simulink model "modelsimulator"  (R2023b)
settings: Solver=VariableStepAuto  StartTime=0.0  StopTime=185  FixedStep=0.0002  RelTol=1e-3
values from neighbouring files (symbols this model uses):
  eta_init = [0 0 0 0 0 0]    [Linearization_validation.m]    (also in ROV_simulation_init.m = [radius 0 0 0 0 -pi/2])
  K_full = lqr(linsysROV_lqr,Q,R)    [ROV_simulation_init.m]
  K_reduced = lqr(linsysROV_lqr_reduced_disc,Q,R)    [ROV_simulation_init.m]
  omega = 0.0174532925*5    (= 0.0872664625)    [ROV_simulation_init.m]
  p = [-125.691529893755	-8.50647884753240	275.922008410927	13.4112646958028	-226.567986780204	-3.28875901062827	118.657519470084	6.62648580653865	14.9826070833980	0.00]    [ROV_simulation_init.m]
  PID_phi = [11.6676, 5.8503, -12.3688, 0.025226,34]    [ROV_simulation_init.m]
  PID_psi = [11.3054, 1.000, -3.8005, 0.087502,30]    [ROV_simulation_init.m]
  PID_theta = [10.2974, 5.9702, -15.653, 0.016423,19]    [ROV_simulation_init.m]
  PID_x = [500.411, 30.5093, -500.8638, 0.032394,110]    [ROV_simulation_init.m]
  PID_y = [500.7275, 20.1075, -500.8002, 0.019369,110]    [ROV_simulation_init.m]
  PID_z = [500.7655, 25.0859, -500.5557, 0.026709,158]    [ROV_simulation_init.m]
  radius = 5    [ROV_simulation_init.m]
  ROV = initializeModelMatrices(m,I,COG,l,w,h,Thrusters)    [CreateGramianROV.m]    (also in CreateROVLin.m = initializeModelMatrices(m, I, COB, dim, BlueROVHeavy); Eigenvalue_tracking.m = initializeModelMatrices(m, I, COB,dim,0); Linearization_validation.m = initializeModelMatrices(m, I, COB,dim,0); ROV_simulation_init.m = initializeModelMatrices(m, Inertia, COB, dim, BlueROVHeavy))
  T_inv = ROV.T'/(ROV.T*ROV.T')    [ROV_simulation_init.m]
  ThrusterVoltage = 14    [ROV_simulation_init.m]
  v_init = [3 0 0 0 0 0]    [Linearization_validation.m]    (also in ROV_simulation_init.m = [omega omega z_rate 0 0 omega])
  z_rate = 0.1    [ROV_simulation_init.m]
libraries: simulink x60
(part 2 of 3)

== system modelsimulator/LQR_full/Subsystem ==
  eta_ref : Inport
  Cos : Trigonometry  Operator=cos
  Demux : Demux  Outputs=6
  Gain : Gain  Gain=1.32
  Gain1 : Gain  Gain=1.32
  Mux : Mux  Inputs=6
  Product : Product
  Sin : Trigonometry
  Sin1 : Trigonometry
  Out1 : Outport
  wires:
  Demux/4 -> Sin/1
  Mux/1 -> Out1/1
  Demux/5 -> Sin1/1, Cos/1
  Gain/1 -> Mux/4
  Product/1 -> Gain/1
  Sin/1 -> Product/1
  Cos/1 -> Product/2
  Gain1/1 -> Mux/5
  Sin1/1 -> Gain1/1
  eta_ref/1 -> Demux/1

== system modelsimulator/LQR_full/Tau_body ==
  Tau : Inport
  Pos : Inport  Port=2
  Demux : Demux  Outputs=6
  Demux1 : Demux  Outputs=6
  InvNED : MATLAB Function  TreatAsAtomicUnit=on
  Mux : Mux  Inputs=6
  Tau_b : Outport
  wires:
  Demux/6 -> InvNED/6(Tau6)
  Demux/5 -> InvNED/5(Tau5)
  Demux/3 -> InvNED/3(Tau3)
  Demux/4 -> InvNED/4(Tau4)
  Demux/2 -> InvNED/2(Tau2)
  Demux/1 -> InvNED/1(Tau1)
  Tau/1 -> Demux/1
  Demux1/1 -> InvNED/7(x)
  Demux1/2 -> InvNED/8(y)
  Demux1/3 -> InvNED/9(z)
  Demux1/4 -> InvNED/10(phi)
  Demux1/5 -> InvNED/11(theta)
  Demux1/6 -> InvNED/12(pzi)
  InvNED/1(x_dot) -> Mux/1
  InvNED/2(y_dot) -> Mux/2
  InvNED/3(z_dot) -> Mux/3
  InvNED/4(phi_dot) -> Mux/4
  InvNED/5(theta_dot) -> Mux/5
  InvNED/6(pzi_dot) -> Mux/6
  Mux/1 -> Tau_b/1
  Pos/1 -> Demux1/1

== system modelsimulator/LQR_reduced/Force allocation ==
  Tau : Inport
  1-D Lookup Table : Lookup_n-D  NumberOfTableDimensions=1  BreakpointsForDimension1=polyval(p,[-1:0.1:1])  Table=[-1:0.1:1]  InternalRulePriority=Speed  RndMeth=Simplest
  Constant7 : Constant  Value=T_inv
  Matrix Multiply : Product  Multiplication=Matrix(*)
  u : Outport
  wires:
  Constant7/1 -> Matrix Multiply/1
  Tau/1 -> Matrix Multiply/2
  Matrix Multiply/1 -> 1-D Lookup Table/1
  1-D Lookup Table/1 -> u/1

== system modelsimulator/LQR_reduced/Subsystem ==
  eta_ref : Inport
  Cos : Trigonometry  Operator=cos
  Demux : Demux  Outputs=6
  Gain : Gain  Gain=1.32
  Gain1 : Gain  Gain=1.32
  Mux : Mux  Inputs=6
  Product : Product
  Sin : Trigonometry
  Sin1 : Trigonometry
  Out1 : Outport
  wires:
  Demux/4 -> Sin/1
  Mux/1 -> Out1/1
  Demux/5 -> Sin1/1, Cos/1
  Gain/1 -> Mux/4
  Product/1 -> Gain/1
  Sin/1 -> Product/1
  Cos/1 -> Product/2
  Gain1/1 -> Mux/5
  Sin1/1 -> Gain1/1
  eta_ref/1 -> Demux/1

== system modelsimulator/PID/Force allocation ==
  Tau : Inport
  1-D Lookup Table : Lookup_n-D  NumberOfTableDimensions=1  BreakpointsForDimension1=polyval(p,[-1:0.1:1])  Table=[-1:0.1:1]  InternalRulePriority=Speed  RndMeth=Simplest
  Constant7 : Constant  Value=T_inv
  Matrix Multiply : Product  Multiplication=Matrix(*)
  u : Outport
  wires:
  Constant7/1 -> Matrix Multiply/1
  Tau/1 -> Matrix Multiply/2
  Matrix Multiply/1 -> 1-D Lookup Table/1
  1-D Lookup Table/1 -> u/1

== system modelsimulator/PID/G1 ==
  ref : Inport
  position : Inport  Port=2
  Derivative : Derivative
  Filter : TransferFcn  Denominator=[Tf 1]
  Gain : Gain  Gain=Kc
  Gain1 : Gain  Gain=Ki
  Gain2 : Gain  Gain=Kd
  Integrator : Integrator  InitialCondition=Arb_pnk  LimitOutput=on  UpperSaturationLimit=umax  LowerSaturationLimit=-umax
  Sum : Sum  Inputs=||+++
  Sum1 : Sum  Inputs=|+-
  u : Outport
  wires:
  Gain2/1 -> Derivative/1
  Gain/1 -> Sum/1
  Derivative/1 -> Sum/3
  Integrator/1 -> Sum/2
  Gain1/1 -> Integrator/1
  Filter/1 -> Gain2/1
  Sum/1 -> u/1
  Sum1/1 -> Gain1/1, Gain/1
  ref/1 -> Sum1/1
  position/1 -> Filter/1, Sum1/2

== system modelsimulator/PID/G2 ==
  ref : Inport
  position : Inport  Port=2
  Derivative : Derivative
  Filter : TransferFcn  Denominator=[Tf 1]
  Gain : Gain  Gain=Kc
  Gain1 : Gain  Gain=Ki
  Gain2 : Gain  Gain=Kd
  Integrator : Integrator  InitialCondition=Arb_pnk  LimitOutput=on  UpperSaturationLimit=umax  LowerSaturationLimit=-umax
  Sum : Sum  Inputs=||+++
  Sum1 : Sum  Inputs=|+-
  u : Outport
  wires:
  position/1 -> Sum1/2, Filter/1
  ref/1 -> Sum1/1
  Sum1/1 -> Gain/1, Gain1/1
  Sum/1 -> u/1
  Filter/1 -> Gain2/1
  Gain1/1 -> Integrator/1
  Integrator/1 -> Sum/2
  Derivative/1 -> Sum/3
  Gain/1 -> Sum/1
  Gain2/1 -> Derivative/1

== system modelsimulator/PID/G3 ==
  ref : Inport
  position : Inport  Port=2
  Derivative : Derivative
  Filter : TransferFcn  Denominator=[Tf 1]
  Gain : Gain  Gain=Kc
  Gain1 : Gain  Gain=Ki
  Gain2 : Gain  Gain=Kd
  Integrator : Integrator  InitialCondition=Arb_pnk  LimitOutput=on  UpperSaturationLimit=umax  LowerSaturationLimit=-umax
  Sum : Sum  Inputs=||+++
  Sum1 : Sum  Inputs=|+-
  u : Outport
  wires:
  Gain2/1 -> Derivative/1
  Gain/1 -> Sum/1
  Derivative/1 -> Sum/3
  Integrator/1 -> Sum/2
  Gain1/1 -> Integrator/1
  Filter/1 -> Gain2/1
  Sum/1 -> u/1
  Sum1/1 -> Gain1/1, Gain/1
  ref/1 -> Sum1/1
  position/1 -> Filter/1, Sum1/2

== system modelsimulator/PID/G4 ==
  ref : Inport
  position : Inport  Port=2
  Derivative : Derivative
  Filter : TransferFcn  Denominator=[Tf 1]
  Gain : Gain  Gain=Kc
  Gain1 : Gain  Gain=Ki
  Gain2 : Gain  Gain=Kd
  Integrator : Integrator  InitialCondition=Arb_pnk  LimitOutput=on  UpperSaturationLimit=umax  LowerSaturationLimit=-umax
  Sum : Sum  Inputs=||+++
  Sum1 : Sum  Inputs=|+-
  u : Outport
  wires:
  position/1 -> Sum1/2, Filter/1
  ref/1 -> Sum1/1
  Sum1/1 -> Gain/1, Gain1/1
  Sum/1 -> u/1
  Filter/1 -> Gain2/1
  Gain1/1 -> Integrator/1
  Integrator/1 -> Sum/2
  Derivative/1 -> Sum/3
  Gain/1 -> Sum/1
  Gain2/1 -> Derivative/1

== system modelsimulator/PID/G5 ==
  ref : Inport
  position : Inport  Port=2
  Derivative : Derivative
  Filter : TransferFcn  Denominator=[Tf 1]
  Gain : Gain  Gain=Kc
  Gain1 : Gain  Gain=Ki
  Gain2 : Gain  Gain=Kd
  Integrator : Integrator  InitialCondition=Arb_pnk  LimitOutput=on  UpperSaturationLimit=umax  LowerSaturationLimit=-umax
  Sum : Sum  Inputs=||+++
  Sum1 : Sum  Inputs=|+-
  u : Outport
  wires:
  Gain2/1 -> Derivative/1
  Gain/1 -> Sum/1
  Derivative/1 -> Sum/3
  Integrator/1 -> Sum/2
  Gain1/1 -> Integrator/1
  Filter/1 -> Gain2/1
  Sum/1 -> u/1
  Sum1/1 -> Gain1/1, Gain/1
  ref/1 -> Sum1/1
  position/1 -> Filter/1, Sum1/2

== system modelsimulator/PID/G6 ==
  ref : Inport
  position : Inport  Port=2
  Derivative : Derivative
  Filter : TransferFcn  Denominator=[Tf 1]
  Gain : Gain  Gain=Kc
  Gain1 : Gain  Gain=Ki
  Gain2 : Gain  Gain=Kd
  Integrator : Integrator  InitialCondition=Arb_pnk  LimitOutput=on  UpperSaturationLimit=umax  LowerSaturationLimit=-umax
  Sum : Sum  Inputs=||+++
  Sum1 : Sum  Inputs=|+-
  u : Outport
  wires:
  position/1 -> Sum1/2, Filter/1
  ref/1 -> Sum1/1
  Sum1/1 -> Gain/1, Gain1/1
  Sum/1 -> u/1
  Filter/1 -> Gain2/1
  Gain1/1 -> Integrator/1
  Integrator/1 -> Sum/2
  Derivative/1 -> Sum/3
  Gain/1 -> Sum/1
  Gain2/1 -> Derivative/1

== system modelsimulator/PID/Tau_body ==
  Tau : Inport
  Pos : Inport  Port=2
  Demux : Demux  Outputs=6
  Demux1 : Demux  Outputs=6
  InvNED : MATLAB Function  TreatAsAtomicUnit=on
  Mux : Mux  Inputs=6
  Tau_b : Outport
  wires:
  Demux/6 -> InvNED/6(Tau6)
  Demux/5 -> InvNED/5(Tau5)
  Demux/3 -> InvNED/3(Tau3)
  Demux/4 -> InvNED/4(Tau4)
  Demux/2 -> InvNED/2(Tau2)
  Demux/1 -> InvNED/1(Tau1)
  Tau/1 -> Demux/1
  Demux1/1 -> InvNED/7(x)
  Demux1/2 -> InvNED/8(y)
  Demux1/3 -> InvNED/9(z)
  Demux1/4 -> InvNED/10(phi)
  Demux1/5 -> InvNED/11(theta)
  Demux1/6 -> InvNED/12(pzi)
  InvNED/1(x_dot) -> Mux/1
  InvNED/2(y_dot) -> Mux/2
  InvNED/3(z_dot) -> Mux/3
  InvNED/4(phi_dot) -> Mux/4
  InvNED/5(theta_dot) -> Mux/5
  InvNED/6(pzi_dot) -> Mux/6
  Mux/1 -> Tau_b/1
  Pos/1 -> Demux1/1

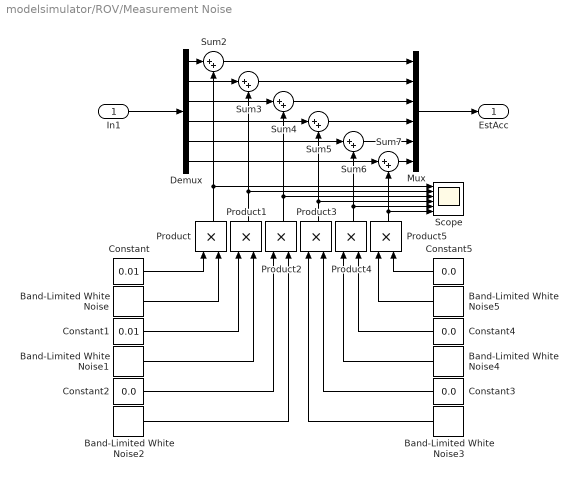
== system modelsimulator/ROV/Measurement Noise ==
  In1 : Inport
  Band-Limited White Noise : simulink/Sources/Band-Limited White Noise  Cov=0.00001  Ts=0.01  seed=[23341]  VectorParams1D=off
  Band-Limited White Noise1 : simulink/Sources/Band-Limited White Noise  Cov=0.00001  Ts=0.01  seed=[23342]  VectorParams1D=off
  Band-Limited White Noise2 : simulink/Sources/Band-Limited White Noise  Cov=0.00001  Ts=0.01  seed=[23343]  VectorParams1D=off
  Band-Limited White Noise3 : simulink/Sources/Band-Limited White Noise  Cov=0.00001  Ts=0.01  seed=[23344]  VectorParams1D=off
  Band-Limited White Noise4 : simulink/Sources/Band-Limited White Noise  Cov=0.00001  Ts=0.01  seed=[23345]  VectorParams1D=off
  Band-Limited White Noise5 : simulink/Sources/Band-Limited White Noise  Cov=0.00001  Ts=0.01  seed=[23346]  VectorParams1D=off
  Constant : Constant  Value=0.01
  Constant1 : Constant  Value=0.01
  Constant{2..5} (4 alike) : Constant  Value=0.0
  Demux : Demux  Outputs=6
  Mux : Mux  Inputs=6
  Product{,1..5} (6 alike) : Product
  Scope : Scope  NumInputPorts=6
  Sum{2..7} (6 alike) : Sum  Inputs=|++
  EstAcc : Outport
  wires:
  Product1/1 -> Scope/2, Sum3/2
  Sum3/1 -> Mux/2
  Demux/2 -> Sum3/1
  Product2/1 -> Scope/3, Sum4/2
  Product4/1 -> Scope/5, Sum6/2
  Band-Limited White Noise5/1 -> Product5/1
  Product5/1 -> Scope/6, Sum7/2
  Constant/1 -> Product/1
  Demux/5 -> Sum6/1
  Band-Limited White Noise1/1 -> Product1/2
  Sum7/1 -> Mux/6
  Product3/1 -> Scope/4, Sum5/2
  Product/1 -> Sum2/2, Scope/1
  Band-Limited White Noise/1 -> Product/2
  Demux/1 -> Sum2/1
  Sum5/1 -> Mux/4
  Sum2/1 -> Mux/1
  Sum4/1 -> Mux/3
  Demux/3 -> Sum4/1
  Band-Limited White Noise3/1 -> Product3/1
  Band-Limited White Noise2/1 -> Product2/2
  Demux/4 -> Sum5/1
  Sum6/1 -> Mux/5
  Mux/1 -> EstAcc/1
  Demux/6 -> Sum7/1
  Band-Limited White Noise4/1 -> Product4/1
  In1/1 -> Demux/1
  Constant1/1 -> Product1/1
  Constant2/1 -> Product2/1
  Constant3/1 -> Product3/2
  Constant4/1 -> Product4/2
  Constant5/1 -> Product5/2

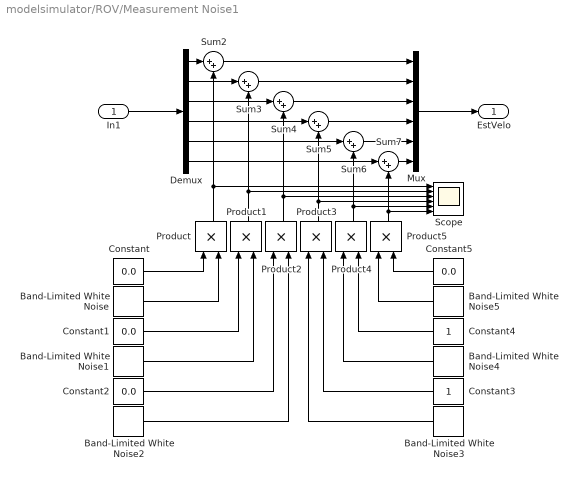
== system modelsimulator/ROV/Measurement Noise1 ==
  In1 : Inport
  Band-Limited White Noise : simulink/Sources/Band-Limited White Noise  Cov=0.00001  Ts=0.01  seed=[23341]  VectorParams1D=off
  Band-Limited White Noise1 : simulink/Sources/Band-Limited White Noise  Cov=0.00001  Ts=0.01  seed=[23342]  VectorParams1D=off
  Band-Limited White Noise2 : simulink/Sources/Band-Limited White Noise  Cov=0.00001  Ts=0.01  seed=[23343]  VectorParams1D=off
  Band-Limited White Noise3 : simulink/Sources/Band-Limited White Noise  Cov=0.00001  Ts=0.01  seed=[23344]  VectorParams1D=off
  Band-Limited White Noise4 : simulink/Sources/Band-Limited White Noise  Cov=0.00001  Ts=0.01  seed=[23345]  VectorParams1D=off
  Band-Limited White Noise5 : simulink/Sources/Band-Limited White Noise  Cov=0.00001  Ts=0.01  seed=[23346]  VectorParams1D=off
  Constant{,1..2,5} (4 alike) : Constant  Value=0.0
  Constant3 : Constant
  Constant4 : Constant
  Demux : Demux  Outputs=6
  Mux : Mux  Inputs=6
  Product{,1..5} (6 alike) : Product
  Scope : Scope  NumInputPorts=6
  Sum{2..7} (6 alike) : Sum  Inputs=|++
  EstVelo : Outport
  wires:
  Constant5/1 -> Product5/2
  Constant4/1 -> Product4/2
  Constant3/1 -> Product3/2
  Constant2/1 -> Product2/1
  Constant1/1 -> Product1/1
  In1/1 -> Demux/1
  Band-Limited White Noise4/1 -> Product4/1
  Demux/6 -> Sum7/1
  Mux/1 -> EstVelo/1
  Sum6/1 -> Mux/5
  Demux/4 -> Sum5/1
  Band-Limited White Noise2/1 -> Product2/2
  Band-Limited White Noise3/1 -> Product3/1
  Demux/3 -> Sum4/1
  Sum4/1 -> Mux/3
  Sum2/1 -> Mux/1
  Sum5/1 -> Mux/4
  Demux/1 -> Sum2/1
  Band-Limited White Noise/1 -> Product/2
  Product/1 -> Scope/1, Sum2/2
  Product3/1 -> Sum5/2, Scope/4
  Sum7/1 -> Mux/6
  Band-Limited White Noise1/1 -> Product1/2
  Demux/5 -> Sum6/1
  Constant/1 -> Product/1
  Product5/1 -> Sum7/2, Scope/6
  Band-Limited White Noise5/1 -> Product5/1
  Product4/1 -> Sum6/2, Scope/5
  Product2/1 -> Sum4/2, Scope/3
  Demux/2 -> Sum3/1
  Sum3/1 -> Mux/2
  Product1/1 -> Sum3/2, Scope/2

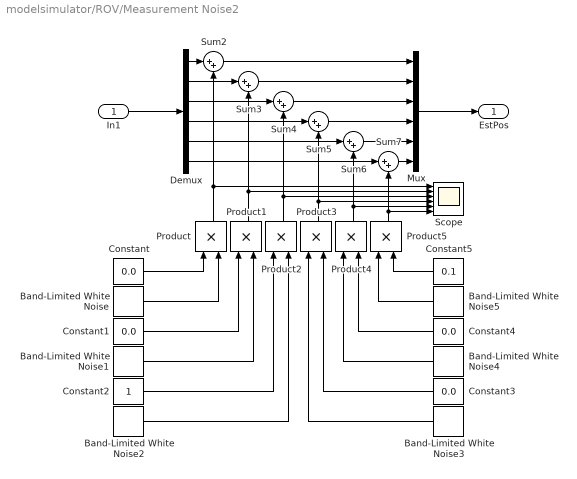
== system modelsimulator/ROV/Measurement Noise2 ==
  In1 : Inport
  Band-Limited White Noise : simulink/Sources/Band-Limited White Noise  Cov=0.00001  Ts=0.01  seed=[23341]  VectorParams1D=off
  Band-Limited White Noise1 : simulink/Sources/Band-Limited White Noise  Cov=0.00001  Ts=0.01  seed=[23342]  VectorParams1D=off
  Band-Limited White Noise2 : simulink/Sources/Band-Limited White Noise  Cov=0.00001  Ts=0.01  seed=[23343]  VectorParams1D=off
  Band-Limited White Noise3 : simulink/Sources/Band-Limited White Noise  Cov=0.00001  Ts=0.01  seed=[23344]  VectorParams1D=off
  Band-Limited White Noise4 : simulink/Sources/Band-Limited White Noise  Cov=0.00001  Ts=0.01  seed=[23345]  VectorParams1D=off
  Band-Limited White Noise5 : simulink/Sources/Band-Limited White Noise  Cov=0.00001  Ts=0.01  seed=[23346]  VectorParams1D=off
  Constant{,1,3..4} (4 alike) : Constant  Value=0.0
  Constant2 : Constant
  Constant5 : Constant  Value=0.1
  Demux : Demux  Outputs=6
  Mux : Mux  Inputs=6
  Product{,1..5} (6 alike) : Product
  Scope : Scope  NumInputPorts=6
  Sum{2..7} (6 alike) : Sum  Inputs=|++
  EstPos : Outport
  wires:
  Product1/1 -> Scope/2, Sum3/2
  Sum3/1 -> Mux/2
  Demux/2 -> Sum3/1
  Product2/1 -> Scope/3, Sum4/2
  Product4/1 -> Scope/5, Sum6/2
  Band-Limited White Noise5/1 -> Product5/1
  Product5/1 -> Scope/6, Sum7/2
  Constant/1 -> Product/1
  Demux/5 -> Sum6/1
  Band-Limited White Noise1/1 -> Product1/2
  Sum7/1 -> Mux/6
  Product3/1 -> Scope/4, Sum5/2
  Product/1 -> Sum2/2, Scope/1
  Band-Limited White Noise/1 -> Product/2
  Demux/1 -> Sum2/1
  Sum5/1 -> Mux/4
  Sum2/1 -> Mux/1
  Sum4/1 -> Mux/3
  Demux/3 -> Sum4/1
  Band-Limited White Noise3/1 -> Product3/1
  Band-Limited White Noise2/1 -> Product2/2
  Demux/4 -> Sum5/1
  Sum6/1 -> Mux/5
  Mux/1 -> EstPos/1
  Demux/6 -> Sum7/1
  Band-Limited White Noise4/1 -> Product4/1
  In1/1 -> Demux/1
  Constant1/1 -> Product1/1
  Constant2/1 -> Product2/1
  Constant3/1 -> Product3/2
  Constant4/1 -> Product4/2
  Constant5/1 -> Product5/2

== system modelsimulator/ROV/NED ==
  velocity : Inport
  position_NED : Inport  Port=2
  Demux : Demux  Outputs=6
  Demux1 : Demux  Outputs=6
  Mux : Mux  Inputs=6
  calcNED : MATLAB Function  TreatAsAtomicUnit=on
  Velocity_NED : Outport
  wires:
  calcNED/2(y_dot) -> Mux/2
  Demux1/5 -> calcNED/11(theta)
  Demux1/4 -> calcNED/10(phi)
  calcNED/1(x_dot) -> Mux/1
  calcNED/3(z_dot) -> Mux/3
  calcNED/5(theta_dot) -> Mux/5
  Demux1/3 -> calcNED/9(z)
  calcNED/4(phi_dot) -> Mux/4
  calcNED/6(pzi_dot) -> Mux/6
  Demux1/2 -> calcNED/8(y)
  Demux/4 -> calcNED/4(p)
  Demux1/6 -> calcNED/12(pzi)
  Demux1/1 -> calcNED/7(x)
  velocity/1 -> Demux/1
  Demux/2 -> calcNED/2(v)
  Demux/1 -> calcNED/1(u)
  Demux/5 -> calcNED/5(q)
  Demux/6 -> calcNED/6(r)
  Demux/3 -> calcNED/3(w)
  position_NED/1 -> Demux1/1
  Mux/1 -> Velocity_NED/1

== system modelsimulator/ROV/NED1 ==
  velocity : Inport
  position_NED : Inport  Port=2
  Demux : Demux  Outputs=6
  Demux1 : Demux  Outputs=6
  Mux : Mux  Inputs=6
  calcNED : MATLAB Function  TreatAsAtomicUnit=on
  Velocity_NED : Outport
  wires:
  Mux/1 -> Velocity_NED/1
  position_NED/1 -> Demux1/1
  Demux/3 -> calcNED/3(w)
  Demux/6 -> calcNED/6(r)
  Demux/5 -> calcNED/5(q)
  Demux/1 -> calcNED/1(u)
  Demux/2 -> calcNED/2(v)
  velocity/1 -> Demux/1
  Demux1/1 -> calcNED/7(x)
  Demux1/6 -> calcNED/12(pzi)
  Demux/4 -> calcNED/4(p)
  Demux1/2 -> calcNED/8(y)
  calcNED/6(pzi_dot) -> Mux/6
  calcNED/4(phi_dot) -> Mux/4
  Demux1/3 -> calcNED/9(z)
  calcNED/5(theta_dot) -> Mux/5
  calcNED/3(z_dot) -> Mux/3
  calcNED/1(x_dot) -> Mux/1
  Demux1/4 -> calcNED/10(phi)
  Demux1/5 -> calcNED/11(theta)
  calcNED/2(y_dot) -> Mux/2

== system modelsimulator/ROV/ROVSubsystem ==
  Velocity : Inport
  Position : Inport  Port=2
  Tau : Inport  Port=3
  Demux : Demux  Outputs=6
  Demux1 : Demux  Outputs=6
  Demux2 : Demux  Outputs=6
  Mux : Mux  Inputs=6
  ROV : MATLAB Function  TreatAsAtomicUnit=on
  Acceleration : Outport
  wires:
  Demux1/1 -> ROV/7(x)
  Demux2/3 -> ROV/3(w)
  ROV/6(r_dot) -> Mux/6
  Demux/2 -> ROV/14(tau2)
  Mux/1 -> Acceleration/1  "Acceleration"
  Demux/4 -> ROV/16(tau4)
  Tau/1 -> Demux/1
  ROV/3(w_dot) -> Mux/3
  ROV/4(p_dot) -> Mux/4
  Demux/6 -> ROV/18(tau6)
  Demux1/2 -> ROV/8(y)
  ROV/1(u_dot) -> Mux/1
  Demux1/3 -> ROV/9(z)
  Demux1/5 -> ROV/11(theta)
  Demux2/6 -> ROV/6(r)
  Demux/1 -> ROV/13(tau1)
  Demux2/4 -> ROV/4(p)
  Velocity/1 -> Demux2/1
  Demux2/5 -> ROV/5(q)
  Demux2/1 -> ROV/1(u)
  Demux/5 -> ROV/17(tau5)
  ROV/5(q_dot) -> Mux/5
  Demux/3 -> ROV/15(tau3)
  Demux1/6 -> ROV/12(pzi)
  Demux1/4 -> ROV/10(phi)
  Demux2/2 -> ROV/2(v)
  ROV/2(v_dot) -> Mux/2
  Position/1 -> Demux1/1

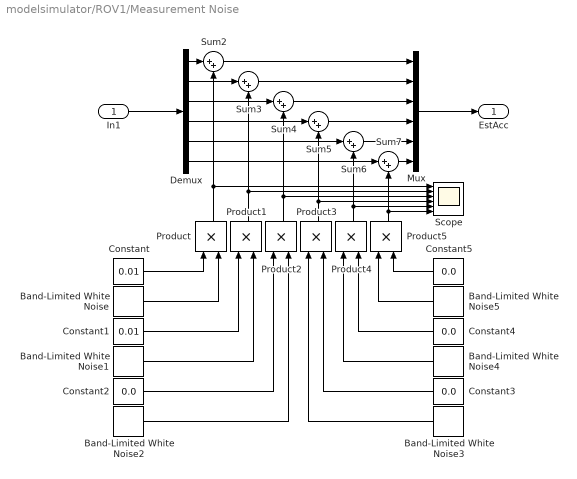
== system modelsimulator/ROV1/Measurement Noise ==
  In1 : Inport
  Band-Limited White Noise : simulink/Sources/Band-Limited White Noise  Cov=0.00001  Ts=0.01  seed=[23341]  VectorParams1D=off
  Band-Limited White Noise1 : simulink/Sources/Band-Limited White Noise  Cov=0.00001  Ts=0.01  seed=[23342]  VectorParams1D=off
  Band-Limited White Noise2 : simulink/Sources/Band-Limited White Noise  Cov=0.00001  Ts=0.01  seed=[23343]  VectorParams1D=off
  Band-Limited White Noise3 : simulink/Sources/Band-Limited White Noise  Cov=0.00001  Ts=0.01  seed=[23344]  VectorParams1D=off
  Band-Limited White Noise4 : simulink/Sources/Band-Limited White Noise  Cov=0.00001  Ts=0.01  seed=[23345]  VectorParams1D=off
  Band-Limited White Noise5 : simulink/Sources/Band-Limited White Noise  Cov=0.00001  Ts=0.01  seed=[23346]  VectorParams1D=off
  Constant : Constant  Value=0.01
  Constant1 : Constant  Value=0.01
  Constant{2..5} (4 alike) : Constant  Value=0.0
  Demux : Demux  Outputs=6
  Mux : Mux  Inputs=6
  Product{,1..5} (6 alike) : Product
  Scope : Scope  NumInputPorts=6
  Sum{2..7} (6 alike) : Sum  Inputs=|++
  EstAcc : Outport
  wires:
  Constant5/1 -> Product5/2
  Constant4/1 -> Product4/2
  Constant3/1 -> Product3/2
  Constant2/1 -> Product2/1
  Constant1/1 -> Product1/1
  In1/1 -> Demux/1
  Band-Limited White Noise4/1 -> Product4/1
  Demux/6 -> Sum7/1
  Mux/1 -> EstAcc/1
  Sum6/1 -> Mux/5
  Demux/4 -> Sum5/1
  Band-Limited White Noise2/1 -> Product2/2
  Band-Limited White Noise3/1 -> Product3/1
  Demux/3 -> Sum4/1
  Sum4/1 -> Mux/3
  Sum2/1 -> Mux/1
  Sum5/1 -> Mux/4
  Demux/1 -> Sum2/1
  Band-Limited White Noise/1 -> Product/2
  Product/1 -> Scope/1, Sum2/2
  Product3/1 -> Sum5/2, Scope/4
  Sum7/1 -> Mux/6
  Band-Limited White Noise1/1 -> Product1/2
  Demux/5 -> Sum6/1
  Constant/1 -> Product/1
  Product5/1 -> Sum7/2, Scope/6
  Band-Limited White Noise5/1 -> Product5/1
  Product4/1 -> Sum6/2, Scope/5
  Product2/1 -> Sum4/2, Scope/3
  Demux/2 -> Sum3/1
  Sum3/1 -> Mux/2
  Product1/1 -> Sum3/2, Scope/2

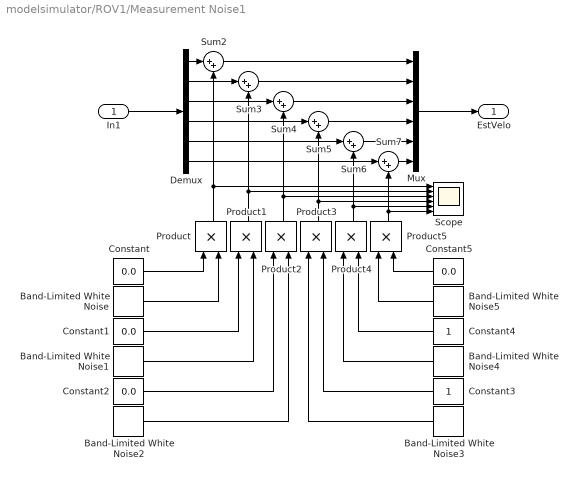
== system modelsimulator/ROV1/Measurement Noise1 ==
  In1 : Inport
  Band-Limited White Noise : simulink/Sources/Band-Limited White Noise  Cov=0.00001  Ts=0.01  seed=[23341]  VectorParams1D=off
  Band-Limited White Noise1 : simulink/Sources/Band-Limited White Noise  Cov=0.00001  Ts=0.01  seed=[23342]  VectorParams1D=off
  Band-Limited White Noise2 : simulink/Sources/Band-Limited White Noise  Cov=0.00001  Ts=0.01  seed=[23343]  VectorParams1D=off
  Band-Limited White Noise3 : simulink/Sources/Band-Limited White Noise  Cov=0.00001  Ts=0.01  seed=[23344]  VectorParams1D=off
  Band-Limited White Noise4 : simulink/Sources/Band-Limited White Noise  Cov=0.00001  Ts=0.01  seed=[23345]  VectorParams1D=off
  Band-Limited White Noise5 : simulink/Sources/Band-Limited White Noise  Cov=0.00001  Ts=0.01  seed=[23346]  VectorParams1D=off
  Constant{,1..2,5} (4 alike) : Constant  Value=0.0
  Constant3 : Constant
  Constant4 : Constant
  Demux : Demux  Outputs=6
  Mux : Mux  Inputs=6
  Product{,1..5} (6 alike) : Product
  Scope : Scope  NumInputPorts=6
  Sum{2..7} (6 alike) : Sum  Inputs=|++
  EstVelo : Outport
  wires:
  Product1/1 -> Scope/2, Sum3/2
  Sum3/1 -> Mux/2
  Demux/2 -> Sum3/1
  Product2/1 -> Scope/3, Sum4/2
  Product4/1 -> Scope/5, Sum6/2
  Band-Limited White Noise5/1 -> Product5/1
  Product5/1 -> Scope/6, Sum7/2
  Constant/1 -> Product/1
  Demux/5 -> Sum6/1
  Band-Limited White Noise1/1 -> Product1/2
  Sum7/1 -> Mux/6
  Product3/1 -> Scope/4, Sum5/2
  Product/1 -> Sum2/2, Scope/1
  Band-Limited White Noise/1 -> Product/2
  Demux/1 -> Sum2/1
  Sum5/1 -> Mux/4
  Sum2/1 -> Mux/1
  Sum4/1 -> Mux/3
  Demux/3 -> Sum4/1
  Band-Limited White Noise3/1 -> Product3/1
  Band-Limited White Noise2/1 -> Product2/2
  Demux/4 -> Sum5/1
  Sum6/1 -> Mux/5
  Mux/1 -> EstVelo/1
  Demux/6 -> Sum7/1
  Band-Limited White Noise4/1 -> Product4/1
  In1/1 -> Demux/1
  Constant1/1 -> Product1/1
  Constant2/1 -> Product2/1
  Constant3/1 -> Product3/2
  Constant4/1 -> Product4/2
  Constant5/1 -> Product5/2

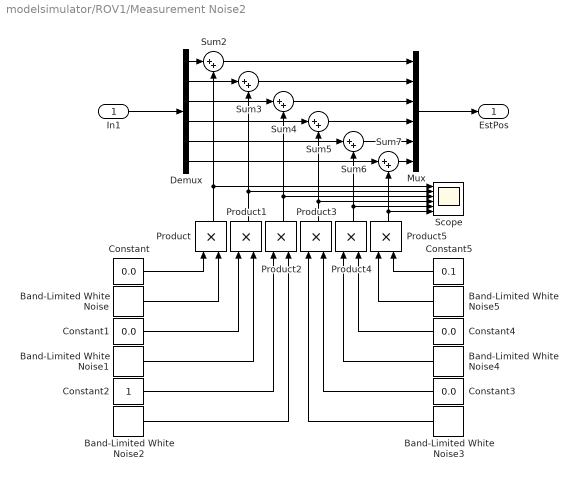
== system modelsimulator/ROV1/Measurement Noise2 ==
  In1 : Inport
  Band-Limited White Noise : simulink/Sources/Band-Limited White Noise  Cov=0.00001  Ts=0.01  seed=[23341]  VectorParams1D=off
  Band-Limited White Noise1 : simulink/Sources/Band-Limited White Noise  Cov=0.00001  Ts=0.01  seed=[23342]  VectorParams1D=off
  Band-Limited White Noise2 : simulink/Sources/Band-Limited White Noise  Cov=0.00001  Ts=0.01  seed=[23343]  VectorParams1D=off
  Band-Limited White Noise3 : simulink/Sources/Band-Limited White Noise  Cov=0.00001  Ts=0.01  seed=[23344]  VectorParams1D=off
  Band-Limited White Noise4 : simulink/Sources/Band-Limited White Noise  Cov=0.00001  Ts=0.01  seed=[23345]  VectorParams1D=off
  Band-Limited White Noise5 : simulink/Sources/Band-Limited White Noise  Cov=0.00001  Ts=0.01  seed=[23346]  VectorParams1D=off
  Constant{,1,3..4} (4 alike) : Constant  Value=0.0
  Constant2 : Constant
  Constant5 : Constant  Value=0.1
  Demux : Demux  Outputs=6
  Mux : Mux  Inputs=6
  Product{,1..5} (6 alike) : Product
  Scope : Scope  NumInputPorts=6
  Sum{2..7} (6 alike) : Sum  Inputs=|++
  EstPos : Outport
  wires:
  Constant5/1 -> Product5/2
  Constant4/1 -> Product4/2
  Constant3/1 -> Product3/2
  Constant2/1 -> Product2/1
  Constant1/1 -> Product1/1
  In1/1 -> Demux/1
  Band-Limited White Noise4/1 -> Product4/1
  Demux/6 -> Sum7/1
  Mux/1 -> EstPos/1
  Sum6/1 -> Mux/5
  Demux/4 -> Sum5/1
  Band-Limited White Noise2/1 -> Product2/2
  Band-Limited White Noise3/1 -> Product3/1
  Demux/3 -> Sum4/1
  Sum4/1 -> Mux/3
  Sum2/1 -> Mux/1
  Sum5/1 -> Mux/4
  Demux/1 -> Sum2/1
  Band-Limited White Noise/1 -> Product/2
  Product/1 -> Scope/1, Sum2/2
  Product3/1 -> Sum5/2, Scope/4
  Sum7/1 -> Mux/6
  Band-Limited White Noise1/1 -> Product1/2
  Demux/5 -> Sum6/1
  Constant/1 -> Product/1
  Product5/1 -> Sum7/2, Scope/6
  Band-Limited White Noise5/1 -> Product5/1
  Product4/1 -> Sum6/2, Scope/5
  Product2/1 -> Sum4/2, Scope/3
  Demux/2 -> Sum3/1
  Sum3/1 -> Mux/2
  Product1/1 -> Sum3/2, Scope/2

== system modelsimulator/ROV1/NED ==
  velocity : Inport
  position_NED : Inport  Port=2
  Demux : Demux  Outputs=6
  Demux1 : Demux  Outputs=6
  Mux : Mux  Inputs=6
  calcNED : MATLAB Function  TreatAsAtomicUnit=on
  Velocity_NED : Outport
  wires:
  Mux/1 -> Velocity_NED/1
  position_NED/1 -> Demux1/1
  Demux/3 -> calcNED/3(w)
  Demux/6 -> calcNED/6(r)
  Demux/5 -> calcNED/5(q)
  Demux/1 -> calcNED/1(u)
  Demux/2 -> calcNED/2(v)
  velocity/1 -> Demux/1
  Demux1/1 -> calcNED/7(x)
  Demux1/6 -> calcNED/12(pzi)
  Demux/4 -> calcNED/4(p)
  Demux1/2 -> calcNED/8(y)
  calcNED/6(pzi_dot) -> Mux/6
  calcNED/4(phi_dot) -> Mux/4
  Demux1/3 -> calcNED/9(z)
  calcNED/5(theta_dot) -> Mux/5
  calcNED/3(z_dot) -> Mux/3
  calcNED/1(x_dot) -> Mux/1
  Demux1/4 -> calcNED/10(phi)
  Demux1/5 -> calcNED/11(theta)
  calcNED/2(y_dot) -> Mux/2

== system modelsimulator/ROV1/NED1 ==
  velocity : Inport
  position_NED : Inport  Port=2
  Demux : Demux  Outputs=6
  Demux1 : Demux  Outputs=6
  Mux : Mux  Inputs=6
  calcNED : MATLAB Function  TreatAsAtomicUnit=on
  Velocity_NED : Outport
  wires:
  calcNED/2(y_dot) -> Mux/2
  Demux1/5 -> calcNED/11(theta)
  Demux1/4 -> calcNED/10(phi)
  calcNED/1(x_dot) -> Mux/1
  calcNED/3(z_dot) -> Mux/3
  calcNED/5(theta_dot) -> Mux/5
  Demux1/3 -> calcNED/9(z)
  calcNED/4(phi_dot) -> Mux/4
  calcNED/6(pzi_dot) -> Mux/6
  Demux1/2 -> calcNED/8(y)
  Demux/4 -> calcNED/4(p)
  Demux1/6 -> calcNED/12(pzi)
  Demux1/1 -> calcNED/7(x)
  velocity/1 -> Demux/1
  Demux/2 -> calcNED/2(v)
  Demux/1 -> calcNED/1(u)
  Demux/5 -> calcNED/5(q)
  Demux/6 -> calcNED/6(r)
  Demux/3 -> calcNED/3(w)
  position_NED/1 -> Demux1/1
  Mux/1 -> Velocity_NED/1

== system modelsimulator/ROV1/ROVSubsystem ==
  Velocity : Inport
  Position : Inport  Port=2
  Tau : Inport  Port=3
  Demux : Demux  Outputs=6
  Demux1 : Demux  Outputs=6
  Demux2 : Demux  Outputs=6
  Mux : Mux  Inputs=6
  ROV : MATLAB Function  TreatAsAtomicUnit=on
  Acceleration : Outport
  wires:
  Position/1 -> Demux1/1
  ROV/2(v_dot) -> Mux/2
  Demux2/2 -> ROV/2(v)
  Demux1/4 -> ROV/10(phi)
  Demux1/6 -> ROV/12(pzi)
  Demux/3 -> ROV/15(tau3)
  ROV/5(q_dot) -> Mux/5
  Demux/5 -> ROV/17(tau5)
  Demux2/1 -> ROV/1(u)
  Demux2/5 -> ROV/5(q)
  Velocity/1 -> Demux2/1
  Demux2/4 -> ROV/4(p)
  Demux/1 -> ROV/13(tau1)
  Demux2/6 -> ROV/6(r)
  Demux1/5 -> ROV/11(theta)
  Demux1/3 -> ROV/9(z)
  ROV/1(u_dot) -> Mux/1
  Demux1/2 -> ROV/8(y)
  Demux/6 -> ROV/18(tau6)
  ROV/4(p_dot) -> Mux/4
  ROV/3(w_dot) -> Mux/3
  Tau/1 -> Demux/1
  Demux/4 -> ROV/16(tau4)
  Mux/1 -> Acceleration/1  "Acceleration"
  Demux/2 -> ROV/14(tau2)
  ROV/6(r_dot) -> Mux/6
  Demux2/3 -> ROV/3(w)
  Demux1/1 -> ROV/7(x)

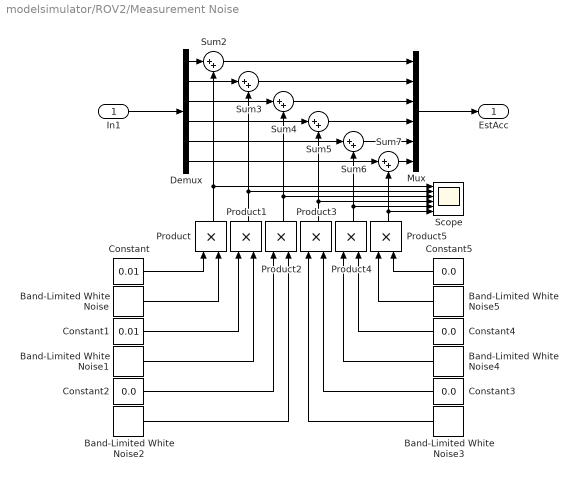
== system modelsimulator/ROV2/Measurement Noise ==
  In1 : Inport
  Band-Limited White Noise : simulink/Sources/Band-Limited White Noise  Cov=0.00001  Ts=0.01  seed=[23341]  VectorParams1D=off
  Band-Limited White Noise1 : simulink/Sources/Band-Limited White Noise  Cov=0.00001  Ts=0.01  seed=[23342]  VectorParams1D=off
  Band-Limited White Noise2 : simulink/Sources/Band-Limited White Noise  Cov=0.00001  Ts=0.01  seed=[23343]  VectorParams1D=off
  Band-Limited White Noise3 : simulink/Sources/Band-Limited White Noise  Cov=0.00001  Ts=0.01  seed=[23344]  VectorParams1D=off
  Band-Limited White Noise4 : simulink/Sources/Band-Limited White Noise  Cov=0.00001  Ts=0.01  seed=[23345]  VectorParams1D=off
  Band-Limited White Noise5 : simulink/Sources/Band-Limited White Noise  Cov=0.00001  Ts=0.01  seed=[23346]  VectorParams1D=off
  Constant : Constant  Value=0.01
  Constant1 : Constant  Value=0.01
  Constant{2..5} (4 alike) : Constant  Value=0.0
  Demux : Demux  Outputs=6
  Mux : Mux  Inputs=6
  Product{,1..5} (6 alike) : Product
  Scope : Scope  NumInputPorts=6
  Sum{2..7} (6 alike) : Sum  Inputs=|++
  EstAcc : Outport
  wires:
  Product1/1 -> Scope/2, Sum3/2
  Sum3/1 -> Mux/2
  Demux/2 -> Sum3/1
  Product2/1 -> Scope/3, Sum4/2
  Product4/1 -> Scope/5, Sum6/2
  Band-Limited White Noise5/1 -> Product5/1
  Product5/1 -> Scope/6, Sum7/2
  Constant/1 -> Product/1
  Demux/5 -> Sum6/1
  Band-Limited White Noise1/1 -> Product1/2
  Sum7/1 -> Mux/6
  Product3/1 -> Scope/4, Sum5/2
  Product/1 -> Sum2/2, Scope/1
  Band-Limited White Noise/1 -> Product/2
  Demux/1 -> Sum2/1
  Sum5/1 -> Mux/4
  Sum2/1 -> Mux/1
  Sum4/1 -> Mux/3
  Demux/3 -> Sum4/1
  Band-Limited White Noise3/1 -> Product3/1
  Band-Limited White Noise2/1 -> Product2/2
  Demux/4 -> Sum5/1
  Sum6/1 -> Mux/5
  Mux/1 -> EstAcc/1
  Demux/6 -> Sum7/1
  Band-Limited White Noise4/1 -> Product4/1
  In1/1 -> Demux/1
  Constant1/1 -> Product1/1
  Constant2/1 -> Product2/1
  Constant3/1 -> Product3/2
  Constant4/1 -> Product4/2
  Constant5/1 -> Product5/2

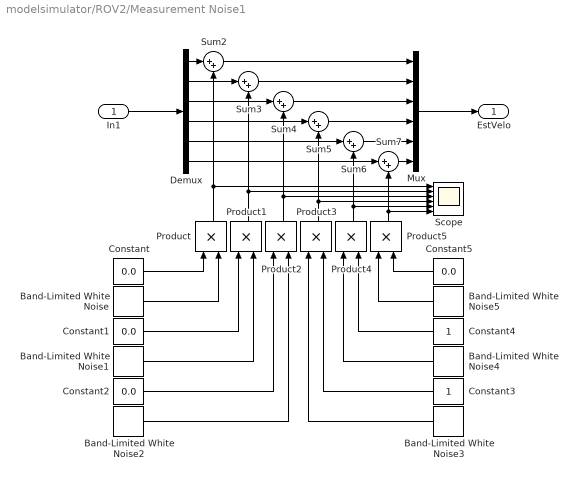
== system modelsimulator/ROV2/Measurement Noise1 ==
  In1 : Inport
  Band-Limited White Noise : simulink/Sources/Band-Limited White Noise  Cov=0.00001  Ts=0.01  seed=[23341]  VectorParams1D=off
  Band-Limited White Noise1 : simulink/Sources/Band-Limited White Noise  Cov=0.00001  Ts=0.01  seed=[23342]  VectorParams1D=off
  Band-Limited White Noise2 : simulink/Sources/Band-Limited White Noise  Cov=0.00001  Ts=0.01  seed=[23343]  VectorParams1D=off
  Band-Limited White Noise3 : simulink/Sources/Band-Limited White Noise  Cov=0.00001  Ts=0.01  seed=[23344]  VectorParams1D=off
  Band-Limited White Noise4 : simulink/Sources/Band-Limited White Noise  Cov=0.00001  Ts=0.01  seed=[23345]  VectorParams1D=off
  Band-Limited White Noise5 : simulink/Sources/Band-Limited White Noise  Cov=0.00001  Ts=0.01  seed=[23346]  VectorParams1D=off
  Constant{,1..2,5} (4 alike) : Constant  Value=0.0
  Constant3 : Constant
  Constant4 : Constant
  Demux : Demux  Outputs=6
  Mux : Mux  Inputs=6
  Product{,1..5} (6 alike) : Product
  Scope : Scope  NumInputPorts=6
  Sum{2..7} (6 alike) : Sum  Inputs=|++
  EstVelo : Outport
  wires:
  Constant5/1 -> Product5/2
  Constant4/1 -> Product4/2
  Constant3/1 -> Product3/2
  Constant2/1 -> Product2/1
  Constant1/1 -> Product1/1
  In1/1 -> Demux/1
  Band-Limited White Noise4/1 -> Product4/1
  Demux/6 -> Sum7/1
  Mux/1 -> EstVelo/1
  Sum6/1 -> Mux/5
  Demux/4 -> Sum5/1
  Band-Limited White Noise2/1 -> Product2/2
  Band-Limited White Noise3/1 -> Product3/1
  Demux/3 -> Sum4/1
  Sum4/1 -> Mux/3
  Sum2/1 -> Mux/1
  Sum5/1 -> Mux/4
  Demux/1 -> Sum2/1
  Band-Limited White Noise/1 -> Product/2
  Product/1 -> Scope/1, Sum2/2
  Product3/1 -> Sum5/2, Scope/4
  Sum7/1 -> Mux/6
  Band-Limited White Noise1/1 -> Product1/2
  Demux/5 -> Sum6/1
  Constant/1 -> Product/1
  Product5/1 -> Sum7/2, Scope/6
  Band-Limited White Noise5/1 -> Product5/1
  Product4/1 -> Sum6/2, Scope/5
  Product2/1 -> Sum4/2, Scope/3
  Demux/2 -> Sum3/1
  Sum3/1 -> Mux/2
  Product1/1 -> Sum3/2, Scope/2

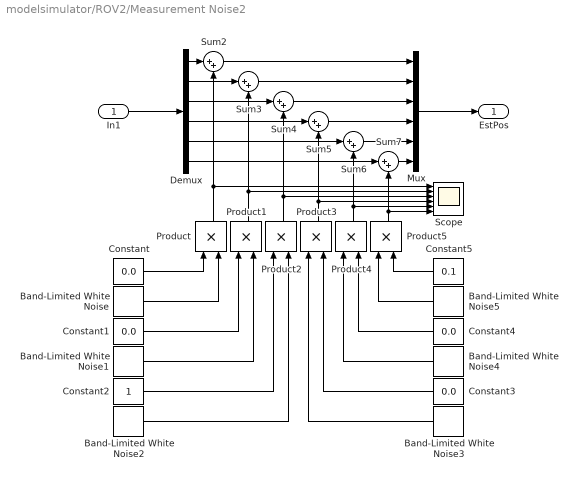
== system modelsimulator/ROV2/Measurement Noise2 ==
  In1 : Inport
  Band-Limited White Noise : simulink/Sources/Band-Limited White Noise  Cov=0.00001  Ts=0.01  seed=[23341]  VectorParams1D=off
  Band-Limited White Noise1 : simulink/Sources/Band-Limited White Noise  Cov=0.00001  Ts=0.01  seed=[23342]  VectorParams1D=off
  Band-Limited White Noise2 : simulink/Sources/Band-Limited White Noise  Cov=0.00001  Ts=0.01  seed=[23343]  VectorParams1D=off
  Band-Limited White Noise3 : simulink/Sources/Band-Limited White Noise  Cov=0.00001  Ts=0.01  seed=[23344]  VectorParams1D=off
  Band-Limited White Noise4 : simulink/Sources/Band-Limited White Noise  Cov=0.00001  Ts=0.01  seed=[23345]  VectorParams1D=off
  Band-Limited White Noise5 : simulink/Sources/Band-Limited White Noise  Cov=0.00001  Ts=0.01  seed=[23346]  VectorParams1D=off
  Constant{,1,3..4} (4 alike) : Constant  Value=0.0
  Constant2 : Constant
  Constant5 : Constant  Value=0.1
  Demux : Demux  Outputs=6
  Mux : Mux  Inputs=6
  Product{,1..5} (6 alike) : Product
  Scope : Scope  NumInputPorts=6
  Sum{2..7} (6 alike) : Sum  Inputs=|++
  EstPos : Outport
  wires:
  Product1/1 -> Scope/2, Sum3/2
  Sum3/1 -> Mux/2
  Demux/2 -> Sum3/1
  Product2/1 -> Scope/3, Sum4/2
  Product4/1 -> Scope/5, Sum6/2
  Band-Limited White Noise5/1 -> Product5/1
  Product5/1 -> Scope/6, Sum7/2
  Constant/1 -> Product/1
  Demux/5 -> Sum6/1
  Band-Limited White Noise1/1 -> Product1/2
  Sum7/1 -> Mux/6
  Product3/1 -> Scope/4, Sum5/2
  Product/1 -> Sum2/2, Scope/1
  Band-Limited White Noise/1 -> Product/2
  Demux/1 -> Sum2/1
  Sum5/1 -> Mux/4
  Sum2/1 -> Mux/1
  Sum4/1 -> Mux/3
  Demux/3 -> Sum4/1
  Band-Limited White Noise3/1 -> Product3/1
  Band-Limited White Noise2/1 -> Product2/2
  Demux/4 -> Sum5/1
  Sum6/1 -> Mux/5
  Mux/1 -> EstPos/1
  Demux/6 -> Sum7/1
  Band-Limited White Noise4/1 -> Product4/1
  In1/1 -> Demux/1
  Constant1/1 -> Product1/1
  Constant2/1 -> Product2/1
  Constant3/1 -> Product3/2
  Constant4/1 -> Product4/2
  Constant5/1 -> Product5/2

== system modelsimulator/ROV2/NED ==
  velocity : Inport
  position_NED : Inport  Port=2
  Demux : Demux  Outputs=6
  Demux1 : Demux  Outputs=6
  Mux : Mux  Inputs=6
  calcNED : MATLAB Function  TreatAsAtomicUnit=on
  Velocity_NED : Outport
  wires:
  calcNED/2(y_dot) -> Mux/2
  Demux1/5 -> calcNED/11(theta)
  Demux1/4 -> calcNED/10(phi)
  calcNED/1(x_dot) -> Mux/1
  calcNED/3(z_dot) -> Mux/3
  calcNED/5(theta_dot) -> Mux/5
  Demux1/3 -> calcNED/9(z)
  calcNED/4(phi_dot) -> Mux/4
  calcNED/6(pzi_dot) -> Mux/6
  Demux1/2 -> calcNED/8(y)
  Demux/4 -> calcNED/4(p)
  Demux1/6 -> calcNED/12(pzi)
  Demux1/1 -> calcNED/7(x)
  velocity/1 -> Demux/1
  Demux/2 -> calcNED/2(v)
  Demux/1 -> calcNED/1(u)
  Demux/5 -> calcNED/5(q)
  Demux/6 -> calcNED/6(r)
  Demux/3 -> calcNED/3(w)
  position_NED/1 -> Demux1/1
  Mux/1 -> Velocity_NED/1

== system modelsimulator/ROV2/NED1 ==
  velocity : Inport
  position_NED : Inport  Port=2
  Demux : Demux  Outputs=6
  Demux1 : Demux  Outputs=6
  Mux : Mux  Inputs=6
  calcNED : MATLAB Function  TreatAsAtomicUnit=on
  Velocity_NED : Outport
  wires:
  Mux/1 -> Velocity_NED/1
  position_NED/1 -> Demux1/1
  Demux/3 -> calcNED/3(w)
  Demux/6 -> calcNED/6(r)
  Demux/5 -> calcNED/5(q)
  Demux/1 -> calcNED/1(u)
  Demux/2 -> calcNED/2(v)
  velocity/1 -> Demux/1
  Demux1/1 -> calcNED/7(x)
  Demux1/6 -> calcNED/12(pzi)
  Demux/4 -> calcNED/4(p)
  Demux1/2 -> calcNED/8(y)
  calcNED/6(pzi_dot) -> Mux/6
  calcNED/4(phi_dot) -> Mux/4
  Demux1/3 -> calcNED/9(z)
  calcNED/5(theta_dot) -> Mux/5
  calcNED/3(z_dot) -> Mux/3
  calcNED/1(x_dot) -> Mux/1
  Demux1/4 -> calcNED/10(phi)
  Demux1/5 -> calcNED/11(theta)
  calcNED/2(y_dot) -> Mux/2

== system modelsimulator/ROV2/ROVSubsystem ==
  Velocity : Inport
  Position : Inport  Port=2
  Tau : Inport  Port=3
  Demux : Demux  Outputs=6
  Demux1 : Demux  Outputs=6
  Demux2 : Demux  Outputs=6
  Mux : Mux  Inputs=6
  ROV : MATLAB Function  TreatAsAtomicUnit=on
  Acceleration : Outport
  wires:
  Demux1/1 -> ROV/7(x)
  Demux2/3 -> ROV/3(w)
  ROV/6(r_dot) -> Mux/6
  Demux/2 -> ROV/14(tau2)
  Mux/1 -> Acceleration/1  "Acceleration"
  Demux/4 -> ROV/16(tau4)
  Tau/1 -> Demux/1
  ROV/3(w_dot) -> Mux/3
  ROV/4(p_dot) -> Mux/4
  Demux/6 -> ROV/18(tau6)
  Demux1/2 -> ROV/8(y)
  ROV/1(u_dot) -> Mux/1
  Demux1/3 -> ROV/9(z)
  Demux1/5 -> ROV/11(theta)
  Demux2/6 -> ROV/6(r)
  Demux/1 -> ROV/13(tau1)
  Demux2/4 -> ROV/4(p)
  Velocity/1 -> Demux2/1
  Demux2/5 -> ROV/5(q)
  Demux2/1 -> ROV/1(u)
  Demux/5 -> ROV/17(tau5)
  ROV/5(q_dot) -> Mux/5
  Demux/3 -> ROV/15(tau3)
  Demux1/6 -> ROV/12(pzi)
  Demux1/4 -> ROV/10(phi)
  Demux2/2 -> ROV/2(v)
  ROV/2(v_dot) -> Mux/2
  Position/1 -> Demux1/1

== system modelsimulator/SMC/Force allocation ==
  Tau : Inport
  1-D Lookup Table : Lookup_n-D  NumberOfTableDimensions=1  BreakpointsForDimension1=polyval(p,[-1:0.1:1])  Table=[-1:0.1:1]  InternalRulePriority=Speed  RndMeth=Simplest
  Constant7 : Constant  Value=T_inv
  Matrix Multiply : Product  Multiplication=Matrix(*)
  u : Outport
  wires:
  Constant7/1 -> Matrix Multiply/1
  Tau/1 -> Matrix Multiply/2
  Matrix Multiply/1 -> 1-D Lookup Table/1
  1-D Lookup Table/1 -> u/1

== system modelsimulator/SMC/SMC_internal ==
  Position : Inport
  Velocity : Inport  Port=2
  Ref : Inport  Port=3
  Ref_d : Inport  Port=4
  Ref_dd : Inport  Port=5
  e_int : Inport  Port=6
  Constant : Constant  Value=0
  Constant1 : Constant  Value=0
  Constant2 : Constant  Value=0
  Demux{,1..5} (6 alike) : Demux  Outputs=6
  Manual Switch : ManualSwitch  CurrentSetting=0
  Manual Switch1 : ManualSwitch  CurrentSetting=0
  Manual Switch2 : ManualSwitch  CurrentSetting=0
  Mux : Mux  Inputs=6
  Position1 : Scope  NumInputPorts=6
  SMC : MATLAB Function  TreatAsAtomicUnit=on
  Tau : Outport
  wires:
  Demux2/1 -> SMC/25(ref_dd1)
  Demux2/2 -> SMC/26(ref_dd2)
  Demux2/3 -> SMC/27(ref_dd3)
  Demux2/4 -> SMC/28(ref_dd4)
  Demux2/5 -> SMC/29(ref_dd5)
  Demux2/6 -> SMC/30(ref_dd6)
  Demux1/1 -> SMC/19(ref_d1)
  Demux1/2 -> SMC/20(ref_d2)
  Demux1/3 -> SMC/21(ref_d3)
  Demux1/4 -> SMC/22(ref_d4)
  Demux1/5 -> SMC/23(ref_d5)
  Demux1/6 -> SMC/24(ref_d6)
  Demux/1 -> SMC/13(ref1)
  Demux/2 -> SMC/14(ref2)
  Demux/3 -> SMC/15(ref3)
  Demux/4 -> SMC/16(ref4)
  Demux/5 -> SMC/17(ref5)
  Demux/6 -> SMC/18(ref6)
  Demux3/1 -> SMC/7(x_d)
  Demux3/2 -> SMC/8(y_d)
  Demux3/3 -> SMC/9(z_d)
  Demux3/4 -> SMC/10(phi_d)
  Demux3/5 -> SMC/11(theta_d)
  Demux3/6 -> SMC/12(pzi_d)
  Demux4/1 -> SMC/1(x)
  Demux4/2 -> SMC/2(y)
  Demux4/3 -> SMC/3(z)
  Demux4/4 -> SMC/4(phi)
  Demux4/5 -> SMC/5(theta)
  Demux4/6 -> SMC/6(pzi)
  Mux/1 -> Tau/1
  Position/1 -> Demux4/1
  Velocity/1 -> Demux3/1
  Ref/1 -> Demux/1
  Ref_d/1 -> Demux1/1
  Ref_dd/1 -> Demux2/1
  Constant/1 -> Manual Switch/1
  SMC/1(Tau_1) -> Manual Switch/2
  Manual Switch/1 -> Mux/1
  SMC/2(Tau_2) -> Manual Switch1/2
  Constant1/1 -> Manual Switch1/1
  Manual Switch1/1 -> Mux/2
  e_int/1 -> Demux5/1
  SMC/7(S_1) -> Position1/1
  SMC/8(S_2) -> Position1/2
  SMC/9(S_3) -> Position1/3
  SMC/10(S_4) -> Position1/4
  SMC/11(S_5) -> Position1/5
  SMC/12(S_6) -> Position1/6
  Demux5/1 -> SMC/31(e_int1)
  Demux5/2 -> SMC/32(e_int2)
  Demux5/3 -> SMC/33(e_int3)
  Demux5/4 -> SMC/34(e_int4)
  Demux5/5 -> SMC/35(e_int5)
  Demux5/6 -> SMC/36(e_int6)
  SMC/5(Tau_5) -> Mux/5
  SMC/4(Tau_4) -> Mux/4
  SMC/3(Tau_3) -> Mux/3
  Manual Switch2/1 -> Mux/6
  SMC/6(Tau_6) -> Manual Switch2/2
  Constant2/1 -> Manual Switch2/1

== system modelsimulator/SMC/Tau_body ==
  Pos : Inport
  Tau : Inport  Port=2
  Demux : Demux  Outputs=6
  Demux1 : Demux  Outputs=6
  InvNED : MATLAB Function  TreatAsAtomicUnit=on
  Mux : Mux  Inputs=6
  Tau_b : Outport
  wires:
  Demux/6 -> InvNED/6(r)
  Demux/5 -> InvNED/5(q)
  Demux/3 -> InvNED/3(w)
  Demux/4 -> InvNED/4(p)
  Demux/2 -> InvNED/2(v)
  Demux/1 -> InvNED/1(u)
  Tau/1 -> Demux/1
  Demux1/1 -> InvNED/7(x)
  Demux1/2 -> InvNED/8(y)
  Demux1/3 -> InvNED/9(z)
  Demux1/4 -> InvNED/10(phi)
  Demux1/5 -> InvNED/11(theta)
  Demux1/6 -> InvNED/12(pzi)
  InvNED/1(x_dot) -> Mux/1
  InvNED/2(y_dot) -> Mux/2
  InvNED/3(z_dot) -> Mux/3
  InvNED/4(phi_dot) -> Mux/4
  InvNED/5(theta_dot) -> Mux/5
  InvNED/6(pzi_dot) -> Mux/6
  Mux/1 -> Tau_b/1
  Pos/1 -> Demux1/1

== system modelsimulator/Step Reference/Subsystem1 ==
  Step : Step  Time=Step_time_1  Before=Init_val  After=New_val  SampleTime=0
  Step1 : Step  Time=Step_time_2  After=New_val  SampleTime=0
  Sum : Sum  Inputs=|+-
  Out1 : Outport
  wires:
  Step1/1 -> Sum/2
  Step/1 -> Sum/1
  Sum/1 -> Out1/1

== system modelsimulator/Step Reference/Subsystem15 ==
  Step : Step  Time=Step_time_1  Before=Init_val  After=New_val  SampleTime=0
  Step1 : Step  Time=Step_time_2  After=New_val  SampleTime=0
  Sum : Sum  Inputs=|+-
  Out1 : Outport
  wires:
  Sum/1 -> Out1/1
  Step/1 -> Sum/1
  Step1/1 -> Sum/2

== system modelsimulator/Step Reference/Subsystem16 ==
  Step : Step  Time=Step_time_1  Before=Init_val  After=New_val  SampleTime=0
  Step1 : Step  Time=Step_time_2  After=New_val  SampleTime=0
  Sum : Sum  Inputs=|+-
  Out1 : Outport
  wires:
  Sum/1 -> Out1/1
  Step/1 -> Sum/1
  Step1/1 -> Sum/2

== system modelsimulator/Step Reference/Subsystem2 ==
  Step : Step  Time=Step_time_1  Before=Init_val  After=New_val  SampleTime=0
  Step1 : Step  Time=Step_time_2  After=New_val  SampleTime=0
  Sum : Sum  Inputs=|+-
  Out1 : Outport
  wires:
  Sum/1 -> Out1/1
  Step/1 -> Sum/1
  Step1/1 -> Sum/2

== system modelsimulator/Step Reference/Subsystem3 ==
  Step : Step  Time=Step_time_1  Before=Init_val  After=New_val  SampleTime=0
  Step1 : Step  Time=Step_time_2  After=New_val  SampleTime=0
  Sum : Sum  Inputs=|+-
  Out1 : Outport
  wires:
  Step1/1 -> Sum/2
  Step/1 -> Sum/1
  Sum/1 -> Out1/1

== system modelsimulator/Step Reference/Subsystem4 ==
  Step : Step  Time=Step_time_1  Before=Init_val  After=New_val  SampleTime=0
  Step1 : Step  Time=Step_time_2  After=New_val  SampleTime=0
  Sum : Sum  Inputs=|+-
  Out1 : Outport
  wires:
  Sum/1 -> Out1/1
  Step/1 -> Sum/1
  Step1/1 -> Sum/2

== system modelsimulator/Step Reference/Subsystem6 ==
  Step : Step  Time=Step_time_1  Before=Init_val  After=New_val  SampleTime=0
  Step1 : Step  Time=Step_time_2  After=New_val  SampleTime=0
  Sum : Sum  Inputs=|+-
  Out1 : Outport
  wires:
  Sum/1 -> Out1/1
  Step/1 -> Sum/1
  Step1/1 -> Sum/2

== system modelsimulator/Step Reference/Subsystem8 ==
  Step : Step  Time=Step_time_1  Before=Init_val  After=New_val  SampleTime=0
  Step1 : Step  Time=Step_time_2  After=New_val  SampleTime=0
  Sum : Sum  Inputs=|+-
  Out1 : Outport
  wires:
  Sum/1 -> Out1/1
  Step/1 -> Sum/1
  Step1/1 -> Sum/2

== system modelsimulator/Step Reference/Subsystem9 ==
  Step : Step  Time=Step_time_1  Before=Init_val  After=New_val  SampleTime=0
  Step1 : Step  Time=Step_time_2  After=New_val  SampleTime=0
  Sum : Sum  Inputs=|+-
  Out1 : Outport
  wires:
  Step1/1 -> Sum/2
  Step/1 -> Sum/1
  Sum/1 -> Out1/1

== system modelsimulator/Thrusters_model1/Subsystem ==
  F : Inport
  Demux : Demux  Outputs=8
  Mux : Mux  Inputs=8
  Transfer Fcn{1..8} (8 alike) : TransferFcn  Numerator=[0 0 -2.1766e+03 2.6574e+06]  Denominator=[1 143.2756 2.9302e+04 2.6574e+06]
  Out1 : Outport
  wires:
  Demux/8 -> Transfer Fcn7/1
  F/1 -> Demux/1
  Mux/1 -> Out1/1
  Transfer Fcn7/1 -> Mux/8
  Demux/7 -> Transfer Fcn1/1
  Transfer Fcn1/1 -> Mux/7
  Transfer Fcn2/1 -> Mux/6
  Demux/6 -> Transfer Fcn2/1
  Demux/5 -> Transfer Fcn3/1
  Transfer Fcn3/1 -> Mux/5
  Transfer Fcn4/1 -> Mux/4
  Demux/4 -> Transfer Fcn4/1
  Demux/3 -> Transfer Fcn5/1
  Transfer Fcn5/1 -> Mux/3
  Demux/2 -> Transfer Fcn6/1
  Transfer Fcn6/1 -> Mux/2
  Demux/1 -> Transfer Fcn8/1
  Transfer Fcn8/1 -> Mux/1

== system modelsimulator/Thrusters_model1/Subsystem1 ==
  F : Inport
  Demux : Demux  Outputs=8
  Mux : Mux  Inputs=8
  Transfer Fcn{1..8} (8 alike) : TransferFcn  Denominator=[1/2 1]
  Out1 : Outport
  wires:
  Demux/8 -> Transfer Fcn7/1
  F/1 -> Demux/1
  Mux/1 -> Out1/1
  Transfer Fcn7/1 -> Mux/8
  Demux/7 -> Transfer Fcn6/1
  Transfer Fcn6/1 -> Mux/7
  Transfer Fcn5/1 -> Mux/6
  Demux/6 -> Transfer Fcn5/1
  Demux/5 -> Transfer Fcn4/1
  Transfer Fcn4/1 -> Mux/5
  Transfer Fcn3/1 -> Mux/4
  Demux/4 -> Transfer Fcn3/1
  Demux/3 -> Transfer Fcn2/1
  Transfer Fcn2/1 -> Mux/3
  Demux/2 -> Transfer Fcn1/1
  Transfer Fcn1/1 -> Mux/2
  Demux/1 -> Transfer Fcn8/1
  Transfer Fcn8/1 -> Mux/1

== system modelsimulator/Thrusters_model2/Subsystem ==
  F : Inport
  Demux : Demux  Outputs=8
  Mux : Mux  Inputs=8
  Transfer Fcn{1..8} (8 alike) : TransferFcn  Numerator=[0 0 -2.1766e+03 2.6574e+06]  Denominator=[1 143.2756 2.9302e+04 2.6574e+06]
  Out1 : Outport
  wires:
  Transfer Fcn5/1 -> Mux/6
  Demux/8 -> Transfer Fcn7/1
  Transfer Fcn2/1 -> Mux/3
  Demux/4 -> Transfer Fcn3/1
  Transfer Fcn3/1 -> Mux/4
  Demux/7 -> Transfer Fcn6/1
  Transfer Fcn4/1 -> Mux/5
  Transfer Fcn6/1 -> Mux/7
  Demux/3 -> Transfer Fcn2/1
  Transfer Fcn7/1 -> Mux/8
  Demux/2 -> Transfer Fcn1/1
  Transfer Fcn1/1 -> Mux/2
  Transfer Fcn8/1 -> Mux/1
  Demux/5 -> Transfer Fcn4/1
  F/1 -> Demux/1
  Demux/1 -> Transfer Fcn8/1
  Demux/6 -> Transfer Fcn5/1
  Mux/1 -> Out1/1

== system modelsimulator/Thrusters_model2/Subsystem1 ==
  F : Inport
  Demux : Demux  Outputs=8
  Mux : Mux  Inputs=8
  Transfer Fcn{1..8} (8 alike) : TransferFcn  Denominator=[1/2 1]
  Out1 : Outport
  wires:
  Demux/8 -> Transfer Fcn7/1
  F/1 -> Demux/1
  Mux/1 -> Out1/1
  Transfer Fcn7/1 -> Mux/8
  Demux/7 -> Transfer Fcn6/1
  Transfer Fcn6/1 -> Mux/7
  Transfer Fcn5/1 -> Mux/6
  Demux/6 -> Transfer Fcn5/1
  Demux/5 -> Transfer Fcn4/1
  Transfer Fcn4/1 -> Mux/5
  Transfer Fcn3/1 -> Mux/4
  Demux/4 -> Transfer Fcn3/1
  Demux/3 -> Transfer Fcn2/1
  Transfer Fcn2/1 -> Mux/3
  Demux/2 -> Transfer Fcn1/1
  Transfer Fcn1/1 -> Mux/2
  Demux/1 -> Transfer Fcn8/1
  Transfer Fcn8/1 -> Mux/1

== system modelsimulator/Thrusters_model3/Subsystem ==
  F : Inport
  Demux : Demux  Outputs=8
  Mux : Mux  Inputs=8
  Transfer Fcn{1..8} (8 alike) : TransferFcn  Numerator=[0 0 -2.1766e+03 2.6574e+06]  Denominator=[1 143.2756 2.9302e+04 2.6574e+06]
  Out1 : Outport
  wires:
  Transfer Fcn5/1 -> Mux/6
  Demux/8 -> Transfer Fcn7/1
  Transfer Fcn2/1 -> Mux/3
  Demux/4 -> Transfer Fcn3/1
  Transfer Fcn3/1 -> Mux/4
  Demux/7 -> Transfer Fcn6/1
  Transfer Fcn4/1 -> Mux/5
  Transfer Fcn6/1 -> Mux/7
  Demux/3 -> Transfer Fcn2/1
  Transfer Fcn7/1 -> Mux/8
  Demux/2 -> Transfer Fcn1/1
  Transfer Fcn1/1 -> Mux/2
  Transfer Fcn8/1 -> Mux/1
  Demux/5 -> Transfer Fcn4/1
  F/1 -> Demux/1
  Demux/1 -> Transfer Fcn8/1
  Demux/6 -> Transfer Fcn5/1
  Mux/1 -> Out1/1

== system modelsimulator/Thrusters_model3/Subsystem2 ==
  F : Inport
  Demux : Demux  Outputs=8
  Mux : Mux  Inputs=8
  Transfer Fcn{1..8} (8 alike) : TransferFcn  Denominator=[1/2 1]
  Out1 : Outport
  wires:
  Transfer Fcn8/1 -> Mux/1
  Demux/1 -> Transfer Fcn8/1
  Transfer Fcn1/1 -> Mux/2
  Demux/2 -> Transfer Fcn1/1
  Transfer Fcn2/1 -> Mux/3
  Demux/3 -> Transfer Fcn2/1
  Demux/4 -> Transfer Fcn3/1
  Transfer Fcn3/1 -> Mux/4
  Transfer Fcn4/1 -> Mux/5
  Demux/5 -> Transfer Fcn4/1
  Demux/6 -> Transfer Fcn5/1
  Transfer Fcn5/1 -> Mux/6
  Transfer Fcn6/1 -> Mux/7
  Demux/7 -> Transfer Fcn6/1
  Transfer Fcn7/1 -> Mux/8
  Mux/1 -> Out1/1
  F/1 -> Demux/1
  Demux/8 -> Transfer Fcn7/1

== matlab function modelsimulator/ROV/NED1/calcNED ==
  data: u input; x_dot output; v input; w input; p input; q input; r input; x input; y input; z input; phi input; theta input; pzi input; y_dot output; z_dot output; phi_dot output; theta_dot output; pzi_dot output
function [x_dot,y_dot,z_dot,phi_dot,theta_dot,pzi_dot] = calcNED(u,v,w,p,q,r,x,y,z,phi,theta,pzi)
%#codegen

%    This function was generated by the Symbolic Math Toolbox version 23.2.
%    06-May-2024 15:56:40

% u = complex(u);  % if required to enforce complex operations
% v = complex(v);  % if required to enforce complex operations
% w = complex(w);  % if required to enforce complex operations
% p = complex(p);  % if required to enforce complex operations
% q = complex(q);  % if required to enforce complex operations
% r = complex(r);  % if required to enforce complex operations
% x = complex(x);  % if required to enforce complex operations
% y = complex(y);  % if required to enforce complex operations
% z = complex(z);  % if required to enforce complex operations
% phi = complex(phi);  % if required to enforce complex operations
% theta = complex(theta);  % if required to enforce complex operations
% pzi = complex(pzi);  % if required to enforce complex operations
t2 = cos(phi);
t3 = cos(pzi);
t4 = cos(theta);
t5 = sin(phi);
t6 = sin(pzi);
t7 = sin(theta);
x_dot = -v.*(t2.*t6-t3.*t5.*t7)+w.*(t5.*t6+t2.*t3.*t7)+t3.*t4.*u;
if nargout > 1
    y_dot = v.*(t2.*t3+t5.*t6.*t7)-w.*(t3.*t5-t2.*t6.*t7)+t4.*t6.*u;
end
if nargout > 2
    z_dot = -t7.*u+t4.*t5.*v+t2.*t4.*w;
end
if nargout > 3
    t8 = tan(theta);
    phi_dot = p+q.*t5.*t8+r.*t2.*t8;
end
if nargout > 4
    theta_dot = q.*t2-r.*t5;
end
if nargout > 5
    t9 = 1.0./t4;
    pzi_dot = q.*t5.*t9+r.*t2.*t9;
end
end

== matlab function modelsimulator/Thrusters_model2/MATLAB Function9 ==
  data: u input; F output; Thruster_voltage input
function F = fcn(u,Thruster_voltage)
if Thruster_voltage == 10
    p = [-92.7173526709009	-4.21942992652299	225.484550494853	8.63193834440817	-201.940923421530	-6.79855430208119	89.8300206612197	5.42728991500474	5.00491978379944	-0.00];
elseif Thruster_voltage == 12
    p = [-102.848572308239	-7.53059973031176	248.621713648981	14.4941570056757	-222.949976245640	-9.82587357024907	101.816137648126	6.80722654001185	7.78963212289893	-0.00];
elseif Thruster_voltage == 14
    p = [-111.940783464042	-6.65861599537878	269.823430407384	13.8659958797022	-243.064927768226	-10.2880091499065	114.063389337106	8.09188399656116	10.6145211900378	-0.00];
elseif Thruster_voltage == 16
    p =  [-148.575215521583	-6.01951344606880	347.062027953365	14.7939725163702	-299.865931981745	-13.0166356354772	134.177990099770	10.1629233711657	12.7092879704266	-0.00];
elseif Thruster_voltage == 18
    p = [-162.288059231193	-9.51335388922301	365.972527557958	19.4413549873700	-302.179637889150	-11.4404685775311	136.049916333434	8.61090564659817	14.1180490642860	-0.00];
elseif Thruster_voltage == 20
    p = [-125.691529893755	-8.50647884753240	275.922008410927	13.4112646958028	-226.567986780204	-3.28875901062827	118.657519470084	6.62648580653865	14.9826070833980	0.00];
else
    p = [0];
end
F = polyval(p,u);
